simulink model "Cruise"  (R2018a)
settings: Solver=VariableStepAuto  StartTime=0.0  StopTime=inf  FixedStep=0.01  RelTol=1e-3  EnableMultiTasking=on
PreLoadFcn:
  | sampleTime = 0.05;
  | 
  | % Vehicle Parameters
  | R = 0.1;
  | L = 0.5;
undefined symbols (not defined in the file): C1, C2, cBW, Waypoint
libraries: cstblocks x3, mobileRoboticsLib x2, dspsrcs4 x1
settings Model: SimulationMode=accelerator  EnablePacing=on  Creator=scastro  LastModifiedBy=shravan
settings DataIOCC: LimitDataPoints=on
settings OptimizationCC: LifeSpan=inf
settings DebuggingCC: AllowSymbolicDim=off  SFUnexpectedBacktrackingDiag=warning  SFNoUnconditionalDefaultTransitionDiag=warning  SFExecutionAtInitializationDiag=none
settings CodeAppCC: StateflowObjectComments=on
settings GRTTargetCC: TargetLangStandard=C89/C90 (ANSI)  GeneratePreprocessorConditionals=Disable all
settings ConfigComp: CovMetricSettings=dw  CovHtmlReporting=on  CovSaveCumulativeToWorkspaceVar=on  CovSaveSingleToWorkspaceVar=on  CovExternalEMLEnable=off  CovSFcnEnable=off
settings SimscapeCC: SimscapeNominalValues="[{\"value\":\"10\",\"unit\":\"V\"},{\"value\":\"1\",\"unit\":\"A\"},{\"value\":\"10\",\"unit\":\"N*m\"},{\"value\":\"10\",\"unit\":\"bar\"},{\"value\":\"100\",\"unit\":\"kJ/kg\"},{\"value\":\"1\",\"unit\":\"kW\"},{\"value\":\"300\",\"unit\":\"K\"},{\"value\":\"100\",\"unit\":\"cm^3/s\"},{\"value\":\"1\",\"unit\":\"kN\"},{\"value\":\"1\",\"unit\":\"g/cm^3\"},{\"value\":\"1\",\"unit\":\"l\"},{\"value\":\"1\",\"unit\":\"cm^2\"},{\"value\":\"60\",\"unit\":\"Hz\"}]"  SimscapeLogType=all  SimscapeLogDataHistory=10000
settings ConfigurationSet: Description=SimMechanics 2G
settings ExplorerConfigSet: InternalSimMechanicsExplorerSettings="<ExplorerConfiguration><canonicalview>default</canonicalview><AnimationSetting><BasePlaybackSpeed>1.0</BasePlaybackSpeed><PlaybackSpeedFactor>1.0</PlaybackSpeedFactor></AnimationSetting><TilePanel><TileInfo><Tiles Columns=\"1\" Count=\"1\" Rows=\"1\"><Column Weight=\"1\"/><Row Weight=\"1\"/><Tile Height=\"1\" Width=\"1\" X=\"0\" Y=\"0\"/></Tiles></TileInfo><SceneInfo><SceneViewer><BGColor><R>0.60000002384185791</R><G>0.60000002384185791</G><B>0.60000002384185791</B></BGColor><Camera><DoPerspective>off</DoPerspective><Position><X>-1.70656042355848525</X><Y>-0.974920623359631922</Y><Z>4.72930454537082046</Z></Position><Center><X>0.552860638431633689</X><Y>1.42025063411503494</Y><Z>1.4843509506914252</Z></Center><Up><X>0.664249622453917166</X><Y>0.300615402055903091</Y><Z>0.684399604848363485</Z></Up><ViewLimDist>1</ViewLimDist><YLim>2.77881717169207398</YLim><XLim>3.55928742670435394</XLim></Camera></SceneViewer></SceneInfo></TilePanel><MechEditorPanel><Cameras/><GfxPanelCameraMap/><VideoCreator><PlaybackSpeedRatio>1.0</PlaybackSpeedRatio><FrameRate>30</FrameRate><VideoFormat>Motion JPEG AVI</VideoFormat><FrameSize>auto</FrameSize></VideoCreator></MechEditorPanel></ExplorerConfiguration>"

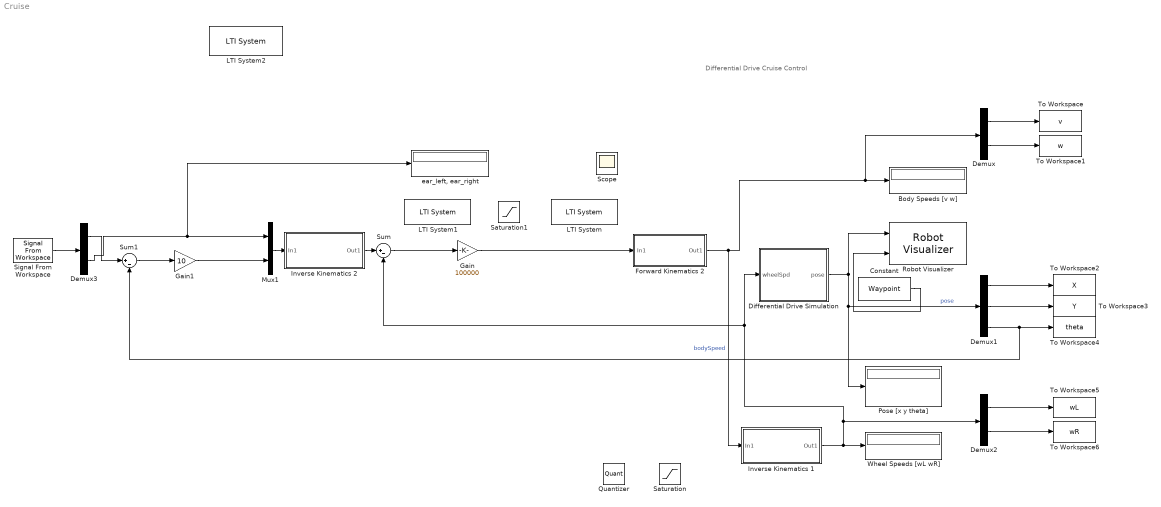
== system Cruise ==
  note: Differential Drive Cruise Control
  Body Speeds [v w] : Display
  Constant : Constant  Value=Waypoint  SampleTime=sampleTime
  Demux : Demux  Outputs=2
  Demux1 : Demux  Outputs=3
  Demux2 : Demux  Outputs=2
  Demux3 : Demux  Outputs=2
  Differential Drive Simulation : Subsystem  AncestorBlock=mobileRoboticsLib/Kinematic Models/Differential Drive/Differential Drive Simulation  OverrideUsingVariant=mode==2  mask(Differential Drive Simulation){wheelRadius=R, wheelBase=L, initX=C1, initY=C2, initAngle=0, Ts=sampleTime}
      mask prompts: wheelRadius "Wheel Radius [m]"; wheelBase "Wheelbase [m]"; initX "Initial X Position [m]"; initY "Initial Y Position [m]"; initAngle "Initial Angle [rad]"; Ts "Sample Time"
      mask help:
      | Simulates the kinematics of a differential drive vehicle from a specified initial pose.
      |
      | Input: Left and right wheel speeds [wL; wR], in rad/s
      |
      | Output: Pose [x; y; theta], in m, m, and rad
      |
      | Set the Sample Time parameter to 0 for continuous-time simulation, or a positive number for discrete-time simulation.
      mask Help: web('matlab:edit mrsDocDifferentialDrive')
      mask Callback Ts:
      | Ts = evalin('base',get_param(gcb,'Ts'));
      | blk = [gcb '/Generic Robot Simulation/Velocity Integrator'];
      | if Ts > 0
      |     set_param(blk,'OverrideUsingVariant','mode==2');
      | else
      |     set_param(blk,'OverrideUsingVariant','mode==1');
      | end
  Forward Kinematics 2 : Subsystem
  Gain : Gain  Gain=100000
  Gain1 : Gain  Gain=10
  Inverse Kinematics 1 : Subsystem
  Inverse Kinematics 2 : Subsystem
  LTI System : cstblocks/LTI System  sys=Plant  IC=[0 0 0 0]
  LTI System1 : cstblocks/LTI System  sys=Controller  IC=[]
  LTI System2 : cstblocks/LTI System  sys=OuterLoop  IC=[]
  Mux1 : Mux  Inputs=2
  Pose [x y theta] : Display
  Quantizer : Quantizer
  Robot Visualizer : mobileRoboticsLib/Environments/Robot Visualizer  Priority=99  robotRadius=1  showTrajectory=on  hasWaypoints=on  hasLidar=off  sensorOffset=[ 0 0 ]  scanAngles=scanAngles  hasObjDetector=off  objDetectorOffset=[ 0, 0 ]  objDetectorAngle=0  objDetectorFOV=pi/4  objDetectorMaxRange=5  objectColors=[ 1, 0, 0; 0, 1, 0; 0, 0, 1 ]  objectMarkers='s'
      settings: SourceProductName=Mobile Robotics Simulation Library
  Saturation : Saturate
  Saturation1 : Saturate  UpperLimit=12  LowerLimit=0
  Scope : Scope
  Signal From Workspace : dspsrcs4/Signal From Workspace  X=Cruise  Ts=cBW  nsamps=1  OutputAfterFinalValue=Holding final value  ignoreOrWarnInputAndFrameLengths=off  OutputFrames=off
  Sum : Sum  Inputs=|+-
  Sum1 : Sum  Inputs=|+-
  To Workspace : ToWorkspace  VariableName=v  SampleTime=-1
  To Workspace1 : ToWorkspace  VariableName=w  SampleTime=-1
  To Workspace2 : ToWorkspace  VariableName=X  SampleTime=sampleTime
  To Workspace3 : ToWorkspace  VariableName=Y  SampleTime=-1
  To Workspace4 : ToWorkspace  VariableName=theta  SampleTime=-1
  To Workspace5 : ToWorkspace  VariableName=wL  SampleTime=-1
  To Workspace6 : ToWorkspace  VariableName=wR  SampleTime=-1
  Wheel Speeds [wL wR] : Display
  "ear_left, ear_right " : Display
  wires:
  Differential Drive Simulation/1(pose) -> Demux1/1, Pose [x y theta]/1, Robot Visualizer/1  "pose"
  Forward Kinematics 2/1(Out1) -> Inverse Kinematics 1/1(In1), Demux/1, Body Speeds [v w]/1  "bodySpeed"
  Demux/1 -> To Workspace/1
  Demux/2 -> To Workspace1/1
  Demux1/1 -> To Workspace2/1
  Demux1/2 -> To Workspace3/1
  Demux2/1 -> To Workspace5/1
  Demux2/2 -> To Workspace6/1
  Constant/1 -> Robot Visualizer/2
  Inverse Kinematics 1/1(Out1) -> Demux2/1, Sum/2, Differential Drive Simulation/1(wheelSpd), Wheel Speeds [wL wR]/1
  Signal From Workspace/1 -> Demux3/1
  Demux3/2 -> "ear_left, ear_right "/1, Mux1/1
  Demux3/1 -> Sum1/1
  Mux1/1 -> Inverse Kinematics 2/1(In1)
  Inverse Kinematics 2/1(Out1) -> Sum/1
  Sum/1 -> Gain/1
  Gain/1 -> Forward Kinematics 2/1(In1)
  Sum1/1 -> Gain1/1
  Gain1/1 -> Mux1/2
  Demux1/3 -> Sum1/2, To Workspace4/1

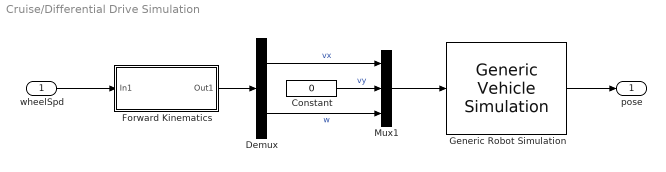
== system Cruise/Differential Drive Simulation ==
  wheelSpd : Inport
  Constant : Constant  Value=0
  Demux : Demux  Outputs=2
  "Forward Kinematics " : Subsystem
  Generic Robot Simulation : mobileRoboticsLib/Utilities/Generic Vehicle Simulation  initX=initX  initY=initY  initAngle=initAngle  Ts=Ts
      link override Velocity Integrator: OverrideUsingVariant=mode==2
      settings: SourceProductName=Mobile Robotics Simulation Toolbox
  Mux1 : Mux  Inputs=3
  pose : Outport
  wires:
  Generic Robot Simulation/1 -> pose/1
  "Forward Kinematics "/1(Out1) -> Demux/1
  wheelSpd/1 -> "Forward Kinematics "/1(In1)
  Constant/1 -> Mux1/2  "vy"
  Demux/2 -> Mux1/3  "w"
  Demux/1 -> Mux1/1  "vx"
  Mux1/1 -> Generic Robot Simulation/1

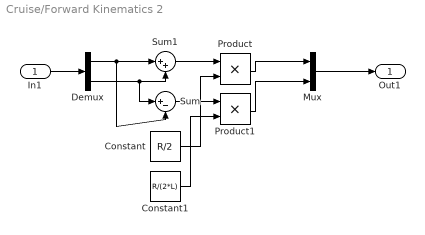
== system Cruise/Forward Kinematics 2 ==
  In1 : Inport
  Constant : Constant  Value=R/2
  Constant1 : Constant  Value=R/(2*L)
  Demux : Demux  Outputs=2
  Mux : Mux  Inputs=2
  Product : Product
  Product1 : Product
  Sum : Sum  Inputs=|+-
  Sum1 : Sum  Inputs=|++
  Out1 : Outport
  wires:
  In1/1 -> Demux/1
  Product1/1 -> Mux/2
  Mux/1 -> Out1/1
  Product/1 -> Mux/1
  Demux/1 -> Sum/2, Sum1/1
  Demux/2 -> Sum/1, Sum1/2
  Sum1/1 -> Product/1
  Constant/1 -> Product/2
  Sum/1 -> Product1/1
  Constant1/1 -> Product1/2

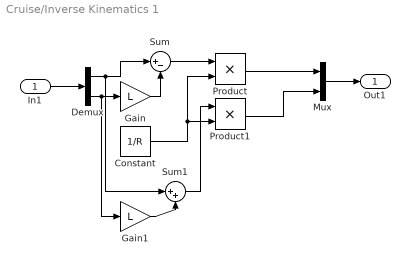
== system Cruise/Inverse Kinematics 1 ==
  In1 : Inport
  Constant : Constant  Value=1/R
  Demux : Demux  Outputs=2
  Gain : Gain  Gain=L
  Gain1 : Gain  Gain=L
  Mux : Mux  Inputs=2
  Product : Product
  Product1 : Product
  Sum : Sum  Inputs=|+-
  Sum1 : Sum  Inputs=|++
  Out1 : Outport
  wires:
  Mux/1 -> Out1/1
  In1/1 -> Demux/1
  Demux/2 -> Gain1/1, Gain/1
  Demux/1 -> Sum1/1, Sum/1
  Gain/1 -> Sum/2
  Sum/1 -> Product/1
  Constant/1 -> Product1/2, Product/2
  Sum1/1 -> Product1/1
  Product/1 -> Mux/1
  Product1/1 -> Mux/2
  Gain1/1 -> Sum1/2

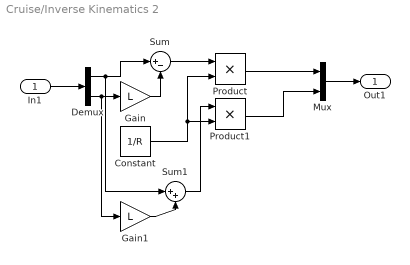
== system Cruise/Inverse Kinematics 2 ==
  In1 : Inport
  Constant : Constant  Value=1/R
  Demux : Demux  Outputs=2
  Gain : Gain  Gain=L
  Gain1 : Gain  Gain=L
  Mux : Mux  Inputs=2
  Product : Product
  Product1 : Product
  Sum : Sum  Inputs=|+-
  Sum1 : Sum  Inputs=|++
  Out1 : Outport
  wires:
  Mux/1 -> Out1/1
  In1/1 -> Demux/1
  Demux/2 -> Gain1/1, Gain/1
  Demux/1 -> Sum1/1, Sum/1
  Gain/1 -> Sum/2
  Sum/1 -> Product/1
  Constant/1 -> Product1/2, Product/2
  Sum1/1 -> Product1/1
  Product/1 -> Mux/1
  Product1/1 -> Mux/2
  Gain1/1 -> Sum1/2

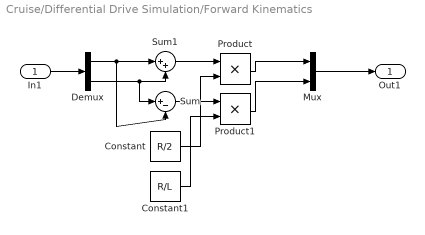
== system Cruise/Differential Drive Simulation/Forward Kinematics  ==
  In1 : Inport
  Constant : Constant  Value=R/2
  Constant1 : Constant  Value=R/L
  Demux : Demux  Outputs=2
  Mux : Mux  Inputs=2
  Product : Product
  Product1 : Product
  Sum : Sum  Inputs=|+-
  Sum1 : Sum  Inputs=|++
  Out1 : Outport
  wires:
  In1/1 -> Demux/1
  Product1/1 -> Mux/2
  Mux/1 -> Out1/1
  Product/1 -> Mux/1
  Demux/1 -> Sum/2, Sum1/1
  Demux/2 -> Sum/1, Sum1/2
  Sum1/1 -> Product/1
  Constant/1 -> Product/2
  Sum/1 -> Product1/1
  Constant1/1 -> Product1/2
